simulink model "pasp_reordertest"  (Simulink 6.2)
settings: Solver=ode45  StartTime=0.0  StopTime=30000  RelTol=1e-3
undefined symbols (not defined in the file or in its folder): iBOB
libraries: xbsIndex_r3 x1464, casper_library x144, xps_library x60
(part 5 of 13)

== system pasp_reordertest/pasp/dist_gbe/reorder ==
  sync : Inport  Port=1  LatchInput=off
  en : Inport  Port=2  LatchInput=off
  din0 : Inport  Port=3  LatchInput=off
  Counter : xbsIndex_r3/Counter  cnt_type=Count Limited  n_bits=14  bin_pt=0  arith_type=Unsigned  start_count=0  cnt_to=12287  cnt_by_val=1  operation=Up  explicit_period=off  period=1  load_pin=off  rst=on  en=on  dbl_ovrd=off  show_param=off  use_rpm=on  gen_core=off
      settings: xl_area=[0, 0, 0, 0, 0, 0, 0]
  Mux : xbsIndex_r3/Mux  inputs=3  precision=Full  arith_type="Signed  (2's comp)"  n_bits=8  bin_pt=2  quantization=Truncate  overflow=Wrap  latency=1  explicit_period=off  period=1  en=off  dbl_ovrd=off  show_param=off  mux_type=off  use_rpm=off  gen_core=off
      settings: xl_area=[0, 0, 0, 0, 0, 0, 0]
  Slice1 : xbsIndex_r3/Slice  mode=Upper Bit Location + Width  nbits=2  bit1=0  base1=MSB of Input  bit0=0  base0=LSB of Input  boolean_output=off  explicit_period=off  period=1  dbl_ovrd=off
  Slice2 : xbsIndex_r3/Slice  mode=Lower Bit Location + Width  nbits=12  bit1=0  base1=MSB of Input  bit0=0  base0=LSB of Input  boolean_output=off  explicit_period=off  period=1  dbl_ovrd=off
  bram0 : xbsIndex_r3/Single Port RAM  depth=4096  initVector=sin(pi*(0:15)/16)  write_mode=Read Before Write  latency=2  init_zero=on  explicit_period=off  period=1  rst=off  init_reg=0  en=off  dbl_ovrd=off  show_param=off  distributed_mem=off  use_rpm=off  gen_core=off
      settings: xl_area=[0, 0, 0, 0, 0, 0, 0]
  delay_d0 : xbsIndex_r3/Delay  latency=2  reg_retiming=off  explicit_period=off  period=1  en=off  accept_only_valid=off  init_zero=on  dbl_ovrd=off  show_param=off
      settings: xl_area=[0, 0, 0, 0, 0, 0, 0]
  delay_din0 : xbsIndex_r3/Delay  latency=3  reg_retiming=off  explicit_period=off  period=1  en=off  accept_only_valid=off  init_zero=on  dbl_ovrd=off  show_param=off
      settings: xl_area=[0, 0, 0, 0, 0, 0, 0]
  delay_map1 : xbsIndex_r3/Delay  latency=1*map_latency  reg_retiming=off  explicit_period=off  period=1  en=off  accept_only_valid=off  init_zero=on  dbl_ovrd=off  show_param=off
      settings: xl_area=[0, 0, 0, 0, 0, 0, 0]
  delay_map2 : xbsIndex_r3/Delay  latency=0*map_latency  reg_retiming=off  explicit_period=off  period=1  en=off  accept_only_valid=off  init_zero=on  dbl_ovrd=off  show_param=off
      settings: xl_area=[0, 0, 0, 0, 0, 0, 0]
  delay_sel : xbsIndex_r3/Delay  latency=2  reg_retiming=off  explicit_period=off  period=1  en=off  accept_only_valid=off  init_zero=on  dbl_ovrd=off  show_param=off
      settings: xl_area=[0, 0, 0, 0, 0, 0, 0]
  delay_valid : xbsIndex_r3/Delay  latency=3  reg_retiming=off  explicit_period=off  period=1  en=off  accept_only_valid=off  init_zero=on  dbl_ovrd=off  show_param=off
      settings: xl_area=[0, 0, 0, 0, 0, 0, 0]
  delay_we : xbsIndex_r3/Delay  latency=2  reg_retiming=off  explicit_period=off  period=1  en=off  accept_only_valid=off  init_zero=on  dbl_ovrd=off  show_param=off
      settings: xl_area=[0, 0, 0, 0, 0, 0, 0]
  map1 : xbsIndex_r3/ROM  depth=4096  initVector=[0 16 32 48 64 80 96 112 128 144 160 176 192 208 224 240 256 272 288 304 320 336 352 368 384 400 416 432 448 464 480 496 512 528 544 560 576 592 608 624 640 656 672 688 704 720 736 752 768 784 800 816 832 848 864 880 896 912 928 944 960 976 992 1008 1024 1040 1056 1072 1088 1104 1120 1136 1152 1168 1184 1200 1216 1232 1248 1264 1280 1296 1312 1328 1344 1360 1376 1392 1408 1424 1440 1456 1472 1488 1504 1520 1536 1552 1568 1584 1600 1616 1632 1648 1664 1680 1696 1712 1728 1744 1760 1776 1792 1808 1824 1840 1856 1872 1888 1904 1920 1936 1952 1968 1984 2000 2016 2032 2048 2064 2080 2096 2112 2128 2144 2160 2176 2192 2208 2224 2240 2256 2272 2288 2304 2320 2336 2352 2368 2384 2400 2416 2432 2448 2464 2480 2496 2512 2528 2544 2560 2576 2592 2608 2624 2640 2656 2672 2688 2704 2720 2736 2752 2768 2784 2800 2816 2832 2848 2864 2880 2896 2912 2928 2944 2960 2976 2992 3008 3024 3040 3056 3072 3088 3104 3120 3136 3152 3168 3184 3200 3216 3232 3248 3264 3280 3296 3312 3328 3344 3360 3376 3392 3408 3424 3440 3456 3472 3488 3504 3520 3536 3552 3568 3584 3600 3616 3632 3648 3664 3680 3696 3712 3728 3744 3760 3776 3792 3808 3824 3840 3856 3872 3888 3904 3920 3936 3952 3968 3984 4000 4016 4032 4048 4064 4080 1 17 33 49 65 81 97 113 129 145 161 177 193 209 225 241 257 273 289 305 321 337 353 369 385 401 417 433 449 465 481 497 513 529 545 561 577 593 609 625 641 657 673 689 705 721 737 753 769 785 801 817 833 849 865 881 897 913 929 945 961 977 993 1009 1025 1041 1057 1073 1089 1105 1121 1137 1153 1169 1185 1201 1217 1233 1249 1265 1281 1297 1313 1329 1345 1361 1377 1393 1409 1425 1441 1457 1473 1489 1505 1521 1537 1553 1569 1585 1601 1617 1633 1649 1665 1681 1697 1713 1729 1745 1761 1777 1793 1809 1825 1841 1857 1873 1889 1905 1921 1937 1953 1969 1985 2001 2017 2033 2049 2065 2081 2097 2113 2129 2145 2161 2177 2193 2209 2225 2241 2257 2273 2289 2305 2321 2337 2353 2369 2385 2401 2417 2433 2449 2465 2481 2497 2513 2529 2545 2561 2577 2593 2609 2625 2641 2657 2673 2689 2705 2721 2737 2753 2769 2785 2801 2817 2833 2849 2865 2881 2897 2913 2929 2945 2961 2977 2993 3009 3025 3041 3057 3073 3089 3105 3121 3137 3153 3169 3185 3201 3217 3233 3249 3265 3281 3297 3313 3329 3345 3361 3377 3393 3409 3425 3441 3457 3473 3489 3505 3521 3537 3553 3569 3585 3601 3617 3633 3649 3665 3681 3697 3713 3729 3745 3761 3777 3793 3809 3825 3841 3857 3873 3889 3905 3921 3937 3953 3969 3985 4001 4017 4033 4049 4065 4081 2 18 34 50 66 82 98 114 130 146 162 178 194 210 226 242 258 274 290 306 322 338 354 370 386 402 418 434 450 466 482 498 514 530 546 562 578 594 610 626 642 658 674 690 706 722 738 754 770 786 802 818 834 850 866 882 898 914 930 946 962 978 994 1010 1026 1042 1058 1074 1090 1106 1122 1138 1154 1170 1186 1202 1218 1234 1250 1266 1282 1298 1314 1330 1346 1362 1378 1394 1410 1426 1442 1458 1474 1490 1506 1522 1538 1554 1570 1586 1602 1618 1634 1650 1666 1682 1698 1714 1730 1746 1762 1778 1794 1810 1826 1842 1858 1874 1890 1906 1922 1938 1954 1970 1986 2002 2018 2034 2050 2066 2082 2098 2114 2130 2146 2162 2178 2194 2210 2226 2242 2258 2274 2290 2306 2322 2338 2354 2370 2386 2402 2418 2434 2450 2466 2482 2498 2514 2530 2546 2562 2578 2594 2610 2626 2642 2658 2674 2690 2706 2722 2738 2754 2770 2786 2802 2818 2834 2850 2866 2882 2898 2914 2930 2946 2962 2978 2994 3010 3026 3042 3058 3074 3090 3106 3122 3138 3154 3170 3186 3202 3218 3234 3250 3266 3282 3298 3314 3330 3346 3362 3378 3394 3410 3426 3442 3458 3474 3490 3506 3522 3538 3554 3570 3586 3602 3618 3634 3650 3666 3682 3698 3714 3730 3746 3762 3778 3794 3810 3826 3842 3858 3874 3890 3906 3922 3938 3954 3970 3986 4002 4018 4034 4050 4066 4082 3 19 35 51 67 83 99 115 131 147 163 179 195 211 227 243 259 275 291 307 323 339 355 371 387 403 419 435 451 467 483 499 515 531 547 563 579 595 611 627 643 659 675 691 707 723 739 755 771 787 803 819 835 851 867 883 899 915 931 947 963 979 995 1011 1027 1043 1059 1075 1091 1107 1123 1139 1155 1171 1187 1203 1219 1235 1251 1267 1283 1299 1315 1331 1347 1363 1379 1395 ...(+15374 chars)]  arith_type=Unsigned  n_bits=12  bin_pt=0  latency=1  init_zero=on  explicit_period=off  period=1  rst=off  init_reg=0  en=off  dbl_ovrd=off  show_param=on  distributed_mem=off  use_rpm=off  gen_core=off
      settings: xl_area=[0, 0, 0, 0, 0, 0, 0]
  map2 : xbsIndex_r3/ROM  depth=4096  initVector=[0 16 32 48 64 80 96 112 128 144 160 176 192 208 224 240 256 272 288 304 320 336 352 368 384 400 416 432 448 464 480 496 512 528 544 560 576 592 608 624 640 656 672 688 704 720 736 752 768 784 800 816 832 848 864 880 896 912 928 944 960 976 992 1008 1024 1040 1056 1072 1088 1104 1120 1136 1152 1168 1184 1200 1216 1232 1248 1264 1280 1296 1312 1328 1344 1360 1376 1392 1408 1424 1440 1456 1472 1488 1504 1520 1536 1552 1568 1584 1600 1616 1632 1648 1664 1680 1696 1712 1728 1744 1760 1776 1792 1808 1824 1840 1856 1872 1888 1904 1920 1936 1952 1968 1984 2000 2016 2032 2048 2064 2080 2096 2112 2128 2144 2160 2176 2192 2208 2224 2240 2256 2272 2288 2304 2320 2336 2352 2368 2384 2400 2416 2432 2448 2464 2480 2496 2512 2528 2544 2560 2576 2592 2608 2624 2640 2656 2672 2688 2704 2720 2736 2752 2768 2784 2800 2816 2832 2848 2864 2880 2896 2912 2928 2944 2960 2976 2992 3008 3024 3040 3056 3072 3088 3104 3120 3136 3152 3168 3184 3200 3216 3232 3248 3264 3280 3296 3312 3328 3344 3360 3376 3392 3408 3424 3440 3456 3472 3488 3504 3520 3536 3552 3568 3584 3600 3616 3632 3648 3664 3680 3696 3712 3728 3744 3760 3776 3792 3808 3824 3840 3856 3872 3888 3904 3920 3936 3952 3968 3984 4000 4016 4032 4048 4064 4080 1 17 33 49 65 81 97 113 129 145 161 177 193 209 225 241 257 273 289 305 321 337 353 369 385 401 417 433 449 465 481 497 513 529 545 561 577 593 609 625 641 657 673 689 705 721 737 753 769 785 801 817 833 849 865 881 897 913 929 945 961 977 993 1009 1025 1041 1057 1073 1089 1105 1121 1137 1153 1169 1185 1201 1217 1233 1249 1265 1281 1297 1313 1329 1345 1361 1377 1393 1409 1425 1441 1457 1473 1489 1505 1521 1537 1553 1569 1585 1601 1617 1633 1649 1665 1681 1697 1713 1729 1745 1761 1777 1793 1809 1825 1841 1857 1873 1889 1905 1921 1937 1953 1969 1985 2001 2017 2033 2049 2065 2081 2097 2113 2129 2145 2161 2177 2193 2209 2225 2241 2257 2273 2289 2305 2321 2337 2353 2369 2385 2401 2417 2433 2449 2465 2481 2497 2513 2529 2545 2561 2577 2593 2609 2625 2641 2657 2673 2689 2705 2721 2737 2753 2769 2785 2801 2817 2833 2849 2865 2881 2897 2913 2929 2945 2961 2977 2993 3009 3025 3041 3057 3073 3089 3105 3121 3137 3153 3169 3185 3201 3217 3233 3249 3265 3281 3297 3313 3329 3345 3361 3377 3393 3409 3425 3441 3457 3473 3489 3505 3521 3537 3553 3569 3585 3601 3617 3633 3649 3665 3681 3697 3713 3729 3745 3761 3777 3793 3809 3825 3841 3857 3873 3889 3905 3921 3937 3953 3969 3985 4001 4017 4033 4049 4065 4081 2 18 34 50 66 82 98 114 130 146 162 178 194 210 226 242 258 274 290 306 322 338 354 370 386 402 418 434 450 466 482 498 514 530 546 562 578 594 610 626 642 658 674 690 706 722 738 754 770 786 802 818 834 850 866 882 898 914 930 946 962 978 994 1010 1026 1042 1058 1074 1090 1106 1122 1138 1154 1170 1186 1202 1218 1234 1250 1266 1282 1298 1314 1330 1346 1362 1378 1394 1410 1426 1442 1458 1474 1490 1506 1522 1538 1554 1570 1586 1602 1618 1634 1650 1666 1682 1698 1714 1730 1746 1762 1778 1794 1810 1826 1842 1858 1874 1890 1906 1922 1938 1954 1970 1986 2002 2018 2034 2050 2066 2082 2098 2114 2130 2146 2162 2178 2194 2210 2226 2242 2258 2274 2290 2306 2322 2338 2354 2370 2386 2402 2418 2434 2450 2466 2482 2498 2514 2530 2546 2562 2578 2594 2610 2626 2642 2658 2674 2690 2706 2722 2738 2754 2770 2786 2802 2818 2834 2850 2866 2882 2898 2914 2930 2946 2962 2978 2994 3010 3026 3042 3058 3074 3090 3106 3122 3138 3154 3170 3186 3202 3218 3234 3250 3266 3282 3298 3314 3330 3346 3362 3378 3394 3410 3426 3442 3458 3474 3490 3506 3522 3538 3554 3570 3586 3602 3618 3634 3650 3666 3682 3698 3714 3730 3746 3762 3778 3794 3810 3826 3842 3858 3874 3890 3906 3922 3938 3954 3970 3986 4002 4018 4034 4050 4066 4082 3 19 35 51 67 83 99 115 131 147 163 179 195 211 227 243 259 275 291 307 323 339 355 371 387 403 419 435 451 467 483 499 515 531 547 563 579 595 611 627 643 659 675 691 707 723 739 755 771 787 803 819 835 851 867 883 899 915 931 947 963 979 995 1011 1027 1043 1059 1075 1091 1107 1123 1139 1155 1171 1187 1203 1219 1235 1251 1267 1283 1299 1315 1331 1347 1363 1379 1395 ...(+15374 chars)]  arith_type=Unsigned  n_bits=12  bin_pt=0  latency=1  init_zero=on  explicit_period=off  period=1  rst=off  init_reg=0  en=off  dbl_ovrd=off  show_param=off  distributed_mem=off  use_rpm=off  gen_core=off
      settings: xl_area=[0, 0, 0, 0, 0, 0, 0]
  post_sync_delay : xbsIndex_r3/Delay  latency=3  reg_retiming=off  explicit_period=off  period=1  en=off  accept_only_valid=off  init_zero=on  dbl_ovrd=off  show_param=off
      settings: xl_area=[0, 0, 0, 0, 0, 0, 0]
  pre_sync_delay : xbsIndex_r3/Delay  latency=2  reg_retiming=off  explicit_period=off  period=1  en=off  accept_only_valid=off  init_zero=on  dbl_ovrd=off  show_param=off
      settings: xl_area=[0, 0, 0, 0, 0, 0, 0]
  sync_delay_en : casper_library/Delays/sync_delay_en  DelayLen=4096
      link override Constant: equ=P=C
      link override Constant1: equ=P=C
      link override Constant2: equ=P=C
      link override Constant3: equ=P=C
  sync_out : Outport
  valid : Outport  Port=2
  dout0 : Outport  Port=3
  wires:
  sync/1 -> Counter/1, pre_sync_delay/1
  en/1 -> Counter/2, sync_delay_en/2, delay_we/1
  Counter/1 -> Slice1/1, Slice2/1
  Slice1/1 -> delay_sel/1
  delay_sel/1 -> Mux/1
  Slice2/1 -> delay_d0/1, map1/1
  delay_d0/1 -> Mux/2
  pre_sync_delay/1 -> sync_delay_en/1
  sync_delay_en/1 -> post_sync_delay/1
  post_sync_delay/1 -> sync_out/1
  delay_we/1 -> delay_valid/1, bram0/3
  delay_valid/1 -> valid/1
  Mux/1 -> bram0/1
  din0/1 -> delay_din0/1
  delay_din0/1 -> bram0/2
  bram0/1 -> dout0/1
  map1/1 -> delay_map1/1, map2/1
  delay_map1/1 -> Mux/3
  map2/1 -> delay_map2/1
  delay_map2/1 -> Mux/4

== system pasp_reordertest/pasp/fft_wideband_real/fft_biplex_real_4x0 ==
  pol1 : Inport  Port=1  LatchInput=off
  pol2 : Inport  Port=2  LatchInput=off
  pol3 : Inport  Port=3  LatchInput=off
  pol4 : Inport  Port=4  LatchInput=off
  sync : Inport  Port=5  LatchInput=off
  shift : Inport  Port=6  LatchInput=off
  bi_real_unscr_4x : Subsystem  mask{FFTSize=3, bram_latency=2}
      mask prompts: FFTSize "Size of FFT (2^?):"; bram_latency "BRAM Latency"
      mask init:
      | blk = gcb;
      | 
      | set_param([blk,'/reorder'],'map', mat2str(bit_reverse(0:2^(FFTSize-1)-1, FFTSize-1)));
      | set_param([blk,'/reorder'],'bram_latency', num2str(bram_latency));
      | set_param([blk,'/reorder1'],'map', mat2str(bit_reverse(2^(FFTSize-1)-1:-1:0, FFTSize-1)));
      | set_param([blk,'/reorder1'],'bram_latency', num2str(bram_latency));
      | set_param([blk,'/reorder2'],'map', mat2str(2^(FFTSize-1)-1:-1:0));
      | set_param([blk,'/reorder2'],'bram_latency', num2str(bram_latency));
  biplex_core : Subsystem  AncestorBlock=casper_library/FFTs/biplex_core  mask(biplex_core){FFTSize=3, BitWidth=18, quantization=Truncate, overflow=Wrap, add_latency=2, mult_latency=3, bram_latency=2}
      mask prompts: FFTSize "Size of FFT: (2^? pnts)"; BitWidth "Bitwidth: (Max Efficiency at 18 bits)"; quantization "Quantization Behavior"; overflow "Overflow Behavior"; add_latency "Add Latency"; mult_latency "Mult Latency"; bram_latency "BRAM Latency"
      mask init:
      | biplex_core_init(gcb,...
      |     'FFTSize', FFTSize,...
      |     'BitWidth', BitWidth,...
      |     'quantization', quantization,...
      |     'overflow', overflow,...
      |     'add_latency', add_latency,...
      |     'mult_latency', mult_latency,...
      |     'bram_latency', bram_latency);
      settings: AttributesFormatString=FFTSize=3
      mask StyleString: edit,edit,popup(Truncate|Round  (unbiased: +/- Inf)|Round  (unbiased: Even Values)),popup(Wrap|Saturate|Error),edit,edit,edit
  ri_to_c : Subsystem
  ri_to_c1 : Subsystem
  pol1_out : Outport
  pol2_out : Outport  Port=2
  pol3_out : Outport  Port=3
  pol4_out : Outport  Port=4
  of : Outport  Port=5
  sync_out : Outport  Port=6
  wires:
  bi_real_unscr_4x/5(sync_out) -> sync_out/1
  bi_real_unscr_4x/4(pol4_out) -> pol4_out/1
  bi_real_unscr_4x/3(pol3_out) -> pol3_out/1
  bi_real_unscr_4x/2(pol2_out) -> pol2_out/1
  bi_real_unscr_4x/1(pol1_out) -> pol1_out/1
  shift/1 -> biplex_core/4(shift)
  sync/1 -> biplex_core/3(sync)
  pol4/1 -> ri_to_c1/2(im)
  ri_to_c1/1(c) -> biplex_core/2(pol2)
  pol3/1 -> ri_to_c1/1(re)
  pol2/1 -> ri_to_c/2(im)
  ri_to_c/1(c) -> biplex_core/1(pol1)
  pol1/1 -> ri_to_c/1(re)
  biplex_core/3(of) -> of/1
  biplex_core/1(out1) -> bi_real_unscr_4x/1(even)
  biplex_core/2(out2) -> bi_real_unscr_4x/2(odd)
  biplex_core/4(sync_out) -> bi_real_unscr_4x/3(sync)
